simulink model "F16_mod_stock"  (R2024b)
settings: Solver=VariableStepAuto  StartTime=0  StopTime=Tend  RelTol=1e-3
values from neighbouring files (symbols this model uses):
  Param = load_F16_params()    [runF16_mod.m]
libraries: aerolibasang x3, shared6dof x1, aerolibatmos2 x1
settings Model: Creator=sherpa  LastModifiedBy=karth
settings SolverCC: AlgebraicLoopSolver=TrustRegion
settings DataIOCC: SaveFormat=StructureWithTime
settings OptimizationCC: BlockReduction=off  DefaultParameterBehavior=Inlined  OptimizeBlockIOStorage=off  BufferReuse=off
settings DebuggingCC: AlgebraicLoopMsg=none  InitInArrayFormatMsg=none
settings ModelReferenceCC: EnableRefExpFcnMdlSchedulingChecks=on
settings RTWCC: GPUComputeCapability=3.5  DLArmComputeVersion=19.05

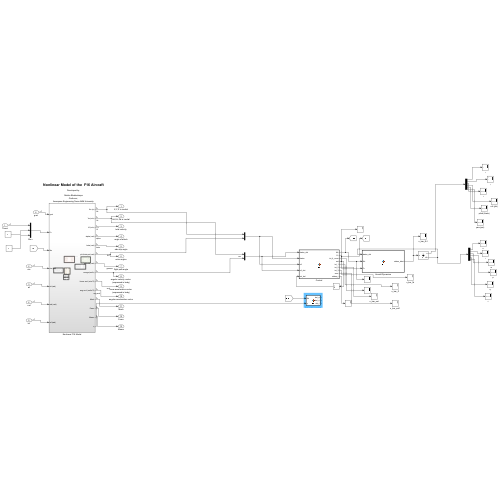
[thumbnail: Simulink's stored preview of the top-level diagram]
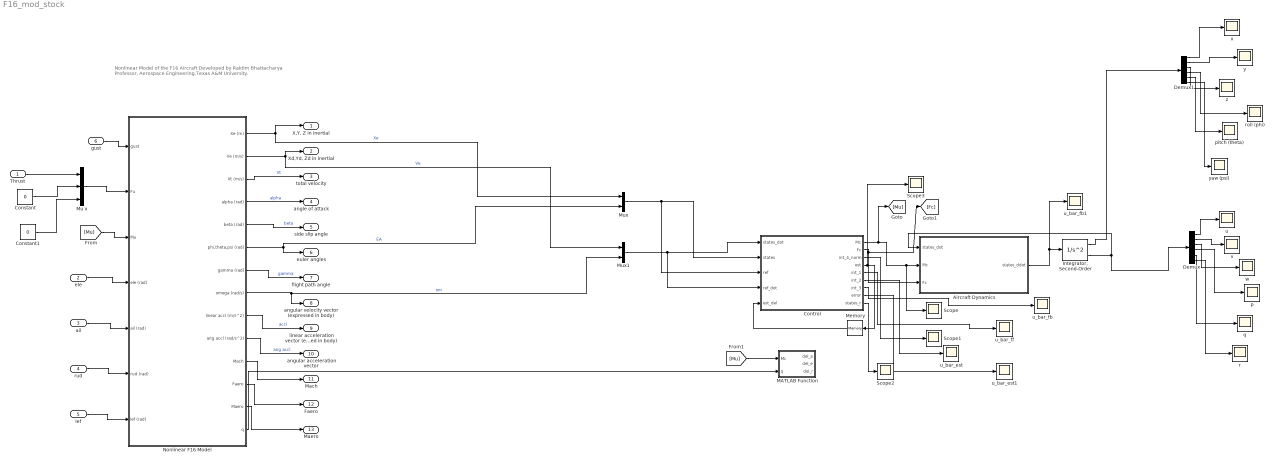
== system F16_mod_stock ==
  note: Nonlinear Model of the F16 Aircraft
      |
      | Developed by
      |
      | Raktim Bhattacharya
      | Professor,
      | Aerospace Engineering,Texas A&M University.
  Thrust : Inport
  ele : Inport  Port=2
  ail : Inport  Port=3
  rud : Inport  Port=4
  lef : Inport  Port=5
  gust : Inport  Port=6
  Aircraft Dynamics : MATLAB Function  TreatAsAtomicUnit=on
  Constant : Constant  Value=0
  Constant1 : Constant  Value=0
  Control : MATLAB Function  TreatAsAtomicUnit=on
  Demux : Demux  Outputs=6
  Demux1 : Demux  Outputs=6
  "Integrator, Second-Order" : SecondOrderIntegrator  ICX=[0;0;0;0;0;0]  ICDXDT=[250;0;0;0;0;0]
  MATLAB Function : MATLAB Function  TreatAsAtomicUnit=on
  Memory : Memory  InitialCondition=[0;0;0]
  Mu x : Mux  Inputs=3
  Mux : Mux  Inputs=2
  Mux1 : Mux  Inputs=2
  Nonlinear F16 Model : Subsystem
  Scope{,1..3} (4 alike) : Scope
  p : Scope
  pitch (theta) : Scope
  q : Scope
  r : Scope
  roll (phi) : Scope
  u : Scope
  u_bar_est : Scope
  u_bar_est1 : Scope
  u_bar_fb : Scope
  u_bar_fb1 : Scope
  u_bar_ff : Scope
  v : Scope
  w : Scope
  x : Scope
  y : Scope
  yaw (psi) : Scope
  z : Scope
  "X,Y, Z in inertial" : Outport
  "Xd,Yd, Zd in inertial" : Outport  Port=2
  total velocity : Outport  Port=3
  angle of attack : Outport  Port=4
  side slip angle : Outport  Port=5
  euler angles : Outport  Port=6
  flight path angle : Outport  Port=7
  angular velocity vector (expressed in body) : Outport  Port=8
  linear acceleration vector (expressed in body) : Outport  Port=9
  angular acceleration vector : Outport  Port=10
  Mach : Outport  Port=11
  Faero : Outport  Port=12
  Maero : Outport  Port=13
  wires:
  Nonlinear F16 Model/1(Xe (m)) -> "X,Y, Z in inertial"/1, Mux/1  "Xe"
  Nonlinear F16 Model/3(Vt (m/s)) -> total velocity/1  "Vt"
  Nonlinear F16 Model/4(alpha (rad)) -> angle of attack/1  "alpha"
  Nonlinear F16 Model/5(beta (rad)) -> side slip angle/1  "beta"
  Nonlinear F16 Model/7(gamma (rad)) -> flight path angle/1  "gamma"
  Nonlinear F16 Model/8(omega (rad/s)) -> angular velocity vector (expressed in body)/1, Mux1/2  "om"
  Nonlinear F16 Model/9(linear accl (m/s^2)) -> linear acceleration vector (expressed in body)/1  "accl"
  Nonlinear F16 Model/6(phi,theta,psi (rad)) -> euler angles/1, Mux/2  "EA"
  Nonlinear F16 Model/2(Ve (m/s)) -> "Xd,Yd, Zd in inertial"/1, Mux1/1  "Ve"
  Nonlinear F16 Model/10(ang accl (rad/s^2)) -> angular acceleration vector/1  "ang accl"
  Nonlinear F16 Model/11(Mach) -> Mach/1
  Thrust/1 -> Mu x/1
  ele/1 -> Nonlinear F16 Model/4(ele (rad))
  rud/1 -> Nonlinear F16 Model/6(rud (rad))
  lef/1 -> Nonlinear F16 Model/7(lef (rad))
  ail/1 -> Nonlinear F16 Model/5(ail (rad))
  gust/1 -> Nonlinear F16 Model/1(gust)
  Nonlinear F16 Model/12(Faero) -> Faero/1
  Nonlinear F16 Model/13(Maero) -> Maero/1
  Demux/3 -> w/1
  Control/7(int_3) -> u_bar_fb/1
  Control/1(Mc) -> [Mu], Scope/1, Aircraft Dynamics/2(Mc)
  Demux1/5 -> pitch (theta)/1
  Control/5(int_1) -> u_bar_ff/1
  Demux/6 -> r/1
  Control/9(states_r) -> Scope2/1
  Control/6(int_2) -> u_bar_est/1
  Aircraft Dynamics/1(states_ddot) -> "Integrator, Second-Order"/1, u_bar_fb1/1
  Demux/1 -> u/1
  Demux1/3 -> z/1
  Demux1/4 -> roll (phi)/1
  Control/3(int_4_norm) -> Scope1/1
  Memory/1 -> Control/5(est_del)
  Demux/2 -> v/1
  Demux/5 -> q/1
  "Integrator, Second-Order"/1 -> Demux1/1
  "Integrator, Second-Order"/2 -> Demux/1, Aircraft Dynamics/1(states_dot)
  Demux1/2 -> y/1
  Control/8(error) -> u_bar_est1/1
  Demux/4 -> p/1
  Demux1/1 -> x/1
  Demux1/6 -> yaw (psi)/1
  Control/4(est) -> Memory/1, Scope3/1
  [Mu] -> Nonlinear F16 Model/3(Mu)
  Control/2(Fc) -> [Fc], Aircraft Dynamics/3(Fc)
  Mux/1 -> Control/3(ref), Control/2(states)
  Mux1/1 -> Control/4(ref_dot), Control/1(states_dot)
  Constant/1 -> Mu x/2
  Mu x/1 -> Nonlinear F16 Model/2(Fu)
  Constant1/1 -> Mu x/3
  Nonlinear F16 Model/14(q) -> MATLAB Function/2(q)
  [Mu] -> MATLAB Function/1(Mc)

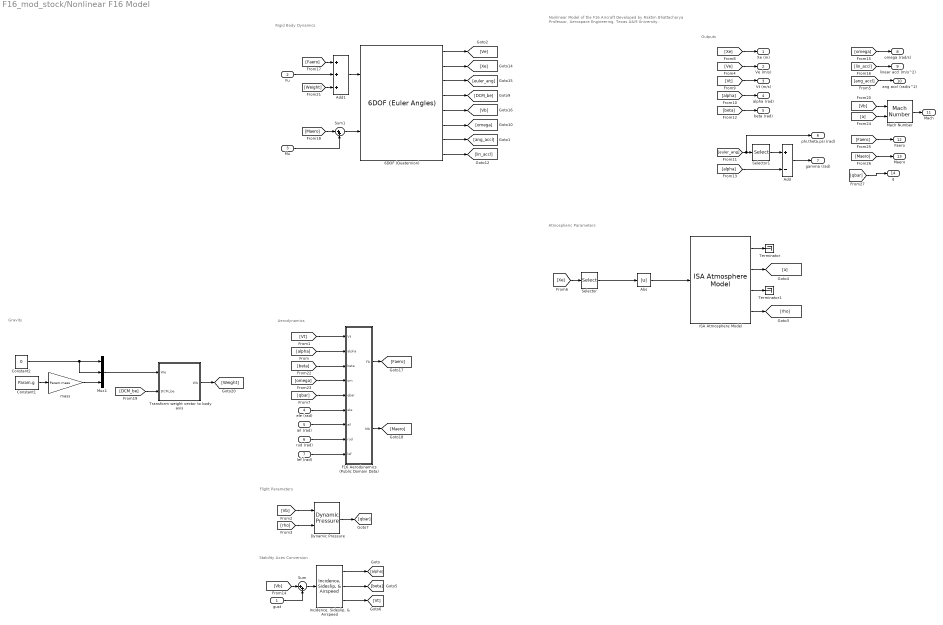
== system F16_mod_stock/Nonlinear F16 Model ==
  note: Gravity
  note: Nonlinear Model of the F16 Aircraft
      |
      | Developed by Raktim Bhattacharya
      | Professor, Aerospace Engineering,
      | Texas A&M University.
  note: Aerodynamics
  note: Outputs
  note: Rigid Body Dynamics
  note: Stability Axes Conversion
  note: Atmospheric Parameters
  note: Flight Parameters
  gust : Inport  PortDimensions=3
  Fu : Inport  Port=2
  Mu : Inport  Port=3  PortDimensions=3
  ele (rad) : Inport  Port=4
  ail (rad) : Inport  Port=5
  rud (rad) : Inport  Port=6
  lef (rad) : Inport  Port=7
  6DOF (Quaternion) : shared6dof/6DOF (Euler Angles)  units=Metric (MKS)  mtype=Fixed  rep=Euler Angles  xme_0=IC.inertial_position  Vm_0=IC.body_velocity  eul_0=IC.euler_angles  pm_0=IC.omega  mass_0=Param.mass  mass_e=0.5  mass_f=2.0  inertia=Param.moi  inertia_e=eye(3)  inertia_f=2*eye(3)  k_quat=1.0  vre_flag=on  abi_flag=off  aMode=0  xme_statename={'Xe', 'Ye', 'Ze'}  Vm_statename={'U', 'v', 'w'}  eul_statename=''  quat_statename={'qr', 'qi', 'qj', 'qk'}  pm_statename={'p', 'q', 'r'}  mass_statename=''
      settings: LibrarySourceBlock=aerolib6dof2/6DOF (Quaternion)
  Abs : Abs  SaturateOnIntegerOverflow=off
  Add : Sum  Inputs=+-
  Add1 : Sum  Inputs=+++
  Constant1 : Constant  Value=Param.g
  Constant2 : Constant  Value=0
  Dynamic Pressure : aerolibasang/Dynamic Pressure
  F16 Aerodynamics (Public Domain Data) : Subsystem
  ISA Atmosphere Model : aerolibatmos2/ISA Atmosphere Model  useExtended=off  action=Warning  custom=off  viscosityOut=off  g=9.80665  gamma=1.4  R=287.0531  L=0.0065  h_trop=11000  h_strat=20000  rho0=1.225  P0=101325  T0=288.15  h0=0  S=110.4  Tref=273.15  muref=1.716e-5
  "Incidence, Sideslip, & Airspeed" : aerolibasang/Incidence, Sideslip, & Airspeed
  Mach Number : aerolibasang/Mach Number
  Mux1 : Mux  Inputs=3
  Selector : Selector  InputPortWidth=3  IndexOptions=Index vector (dialog)  Indices=3  OutputSizes=1
  Selector1 : Selector  InputPortWidth=3  IndexOptions=Index vector (dialog)  Indices=2  OutputSizes=1
  Sum : Sum  Inputs=|++
  Sum1 : Sum  Inputs=|++
  Terminator : Terminator
  Terminator1 : Terminator
  Transform weight vector to body axis : MATLAB Function  TreatAsAtomicUnit=on
  mass : Gain  Gain=Param.mass
  Xe (m) : Outport
  Ve (m/s) : Outport  Port=2
  Vt (m/s) : Outport  Port=3
  alpha (rad) : Outport  Port=4
  beta (rad) : Outport  Port=5
  phi,theta,psi (rad) : Outport  Port=6
  gamma (rad) : Outport  Port=7
  omega (rad/s) : Outport  Port=8
  linear accl (m/s^2) : Outport  Port=9
  ang accl (rad/s^2) : Outport  Port=10
  Mach : Outport  Port=11
  Faero : Outport  Port=12
  Maero : Outport  Port=13
  q : Outport  Port=14
  wires:
  [Xe] -> Selector/1
  [beta] -> beta (rad)/1
  "Incidence, Sideslip, & Airspeed"/3 -> [Vt]
  ISA Atmosphere Model/3 -> Terminator1/1
  ISA Atmosphere Model/1 -> Terminator/1
  ISA Atmosphere Model/4 -> [rho]
  [rho] -> Dynamic Pressure/2
  [lin_accl] -> linear accl (m/s^2)/1
  [alpha] -> alpha (rad)/1
  ISA Atmosphere Model/2 -> [a]
  [Vb] -> Dynamic Pressure/1
  Add/1 -> gamma (rad)/1
  [Vt] -> Vt (m/s)/1
  "Incidence, Sideslip, & Airspeed"/2 -> [beta]
  Selector1/1 -> Add/1
  "Incidence, Sideslip, & Airspeed"/1 -> [alpha]
  Selector/1 -> Abs/1
  [alpha] -> Add/2
  [euler_ang] -> phi,theta,psi (rad)/1, Selector1/1
  [omega] -> omega (rad/s)/1
  Dynamic Pressure/1 -> [qbar]
  [Xe] -> Xe (m)/1
  Constant1/1 -> mass/1
  mass/1 -> Mux1/3
  Mux1/1 -> Transform weight vector to body axis/1(We)
  Transform weight vector to body axis/1(Wb) -> [Weight]
  [DCM_be] -> Transform weight vector to body axis/2(DCM_be)
  Constant2/1 -> Mux1/2, Mux1/1
  [Faero] -> Add1/1
  Fu/1 -> Add1/2
  [Weight] -> Add1/3
  Add1/1 -> 6DOF (Quaternion)/1
  [Vb] -> Sum/1
  Sum/1 -> "Incidence, Sideslip, & Airspeed"/1
  gust/1 -> Sum/2
  [Maero] -> Sum1/1
  Mu/1 -> Sum1/2
  6DOF (Quaternion)/1 -> [Ve]
  6DOF (Quaternion)/2 -> [Xe]
  6DOF (Quaternion)/3 -> [euler_ang]
  6DOF (Quaternion)/4 -> [DCM_be]
  6DOF (Quaternion)/5 -> [Vb]
  6DOF (Quaternion)/6 -> [omega]
  6DOF (Quaternion)/7 -> [ang_accl]
  6DOF (Quaternion)/8 -> [lin_accl]
  [Ve] -> Ve (m/s)/1
  [ang_accl] -> ang accl (rad/s^2)/1
  [Vb] -> Mach Number/1
  [a] -> Mach Number/2
  Mach Number/1 -> Mach/1
  F16 Aerodynamics (Public Domain Data)/1(Fb) -> [Faero]
  Sum1/1 -> 6DOF (Quaternion)/2
  F16 Aerodynamics (Public Domain Data)/2(Mb) -> [Maero]
  [Vt] -> F16 Aerodynamics (Public Domain Data)/1(Vt)
  [alpha] -> F16 Aerodynamics (Public Domain Data)/2(alpha)
  [beta] -> F16 Aerodynamics (Public Domain Data)/3(beta)
  [omega] -> F16 Aerodynamics (Public Domain Data)/4(om)
  [qbar] -> F16 Aerodynamics (Public Domain Data)/5(qbar)
  ele (rad)/1 -> F16 Aerodynamics (Public Domain Data)/6(ele)
  ail (rad)/1 -> F16 Aerodynamics (Public Domain Data)/7(ail)
  rud (rad)/1 -> F16 Aerodynamics (Public Domain Data)/8(rud)
  lef (rad)/1 -> F16 Aerodynamics (Public Domain Data)/9(lef)
  Abs/1 -> ISA Atmosphere Model/1
  [Faero] -> Faero/1
  [Maero] -> Maero/1
  [qbar] -> q/1

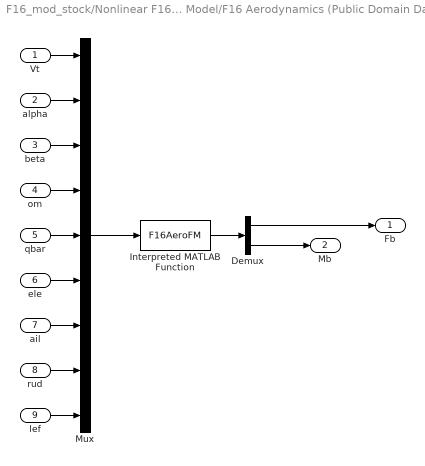
== system F16_mod_stock/Nonlinear F16 Model/F16 Aerodynamics (Public Domain Data) ==
  Vt : Inport
  alpha : Inport  Port=2
  beta : Inport  Port=3
  om : Inport  Port=4
  qbar : Inport  Port=5
  ele : Inport  Port=6
  ail : Inport  Port=7
  rud : Inport  Port=8
  lef : Inport  Port=9
  Demux : Demux  Outputs=2
  Interpreted MATLAB Function : MATLABFcn  MATLABFcn=F16AeroFM  OutputDimensions=6
  Mux : Mux  Inputs=9
  Fb : Outport  PortDimensions=3
  Mb : Outport  Port=2  PortDimensions=3
  wires:
  om/1 -> Mux/4
  beta/1 -> Mux/3
  qbar/1 -> Mux/5
  alpha/1 -> Mux/2
  ele/1 -> Mux/6
  Vt/1 -> Mux/1
  ail/1 -> Mux/7
  rud/1 -> Mux/8
  lef/1 -> Mux/9
  Mux/1 -> Interpreted MATLAB Function/1
  Demux/1 -> Fb/1
  Demux/2 -> Mb/1
  Interpreted MATLAB Function/1 -> Demux/1

== matlab function F16_mod_stock/Nonlinear F16 Model/Transform weight vector to body axis ==
  data: We input; Wb output; DCM_be input
function Wb = fcn(We,DCM_be)
Wb = DCM_be*We; % Weight in body coordinate system. DCM_be is correct, no need for transpose. They must have fixed it in this version.

== matlab function F16_mod_stock/Aircraft Dynamics ==
  data: states_dot input; states_ddot output; Mc input; Fc input
function states_ddot  = fcn(states_dot,Mc,Fc)

% phi, theta , psi == roll_rate, pitch_rate, yaw_rate
theta = 0; % Placeholder angle (pitch) in radians
phi = 0; 

m_aircraft = 24000;
l_aircraft = 17.2;
wingspan = 11.8;
wing_area = 39.9;
wing_width = 4.4;
m_load = 1000;
r_load = 0.3;
n = 4;
wing_mass = 0.12 * m_aircraft;  % this is the combined mass of both wings
r_fuselage = 1.5;
wingspan_new = wingspan - r_fuselage *  2;
m_sym = m_aircraft + n * m_load;
m_asym = m_aircraft + (n-1) * m_load;
%m_aircraft_prime = m_aircraft - m_load; % KR

I_fuselage_origin = 0.5 * (m_aircraft - wing_mass) * r_fuselage.^2;
I_wings = 2 * (1/12) * (wing_mass) * (2 * wing_width.^2);
I_load = n * ((0.5 * m_load * r_load.^2) + (m_load * wing_width.^2));
I_sym = I_fuselage_origin + I_wings + I_load;
cg_x_sym = 0;
cg_y_sym = 0;
cg_z_sym = 0;
cg_shift = (m_aircraft * 0 + (n/2)*m_load - (n/2-1)*m_load)/m_asym;
g = 9.81000;

I_xx_asym = 1.5e4; 
I_yy_asym = 2.0e4;
I_zz_asym = 2.5e4;
I_asym = diag([I_xx_asym, I_yy_asym, I_zz_asym]); % Diagonal terms (kg·m²)

I_xz_asym = 0.02 * I_xx_asym; % Small cross-term (2% of I_xx)
I_yz_asym = 0.02 * I_yy_asym; 
I_xy_asym = 0.02 * I_zz_asym; 

%I_prime = 0; % KR

Zcm = 0.1; 
Ycm = 0.2;
Xcm = 0.15;

% theta = [p q r]^T
% omega = [u v w]^T

p = states_dot(1);
q = states_dot(2);
r = states_dot(3);
u = states_dot(4);
v = states_dot(5);
w = states_dot(6);

Ms = [0;0;0];
Fx = 0;
Fy = 0;
Fz = 0;
Fs = [Fx;Fy;Fz];

A = [0 -m_asym*Zcm m_asym*Ycm; m_asym*Zcm 0 -m_asym*Xcm; -m_asym*Ycm m_asym*Xcm 0];

F1_t = -(q*w) + r*v + (q.^2 + r.^2)*Xcm - (p*q*Ycm) - (r*p*Zcm) + (1/m_asym)*Fx;
F2_t = -(r*u) + p*w + (r.^2 + p.^2)*Ycm - (p*q*Xcm) - (q*r*Zcm) + (1/m_asym)*Fy;
F3_t = -(p*v) + q*u + (p.^2 + q.^2)*Zcm - (r*p*Xcm) - q*r*Ycm + (1/m_asym)*Fz;
F=[F1_t;F2_t;F3_t];

M1_t = I_xz_asym*p*q + (I_yy_asym-I_zz_asym)*q*r - I_xy_asym*r*p + I_yz_asym*(q.^2-r.^2) + m_asym*(q*u - p*v)*Ycm + m_asym*(r*u-p*w)*Zcm + (-Zcm)*m_asym*g*cos(theta)*sin(phi) + Ycm*m_asym*g*cos(theta)*cos(phi);
M2_t = (-I_yz_asym)*p*q + I_xy_asym*q*r + (I_zz_asym-I_xx_asym)*r*p + I_xz_asym*(r.^2-p.^2) + m_asym*(p*v - q*u)*Xcm + m_asym*(r*v-q*w)*Zcm + (-Zcm)*m_asym*g*sin(theta) - Xcm*m_asym*g*cos(theta)*cos(phi);
M3_t = (I_xx_asym-I_yy_asym)*p*q - I_xz_asym*q*r - I_yz_asym*r*p + I_xy_asym*(p.^2-q.^2) + m_asym*(p*w - r*u)*Xcm + m_asym*(q*w-r*v)*Ycm + Ycm*m_asym*g*sin(theta) + Xcm*m_asym*g*cos(theta)*sin(phi);

Mi = [M1_t;M2_t;M3_t];

Fx = Fc(1);
Fy = Fc(2);
Fz = Fc(3);

u_dot = -q*w + r*v - g*sin(theta) + (1/m_sym)*Fx;
v_dot = -r*u + p*w + g*cos(theta)*sin(phi) + (1/m_sym)*Fy;
w_dot = -p*v + q*u + g*cos(theta)*cos(phi) + (1/m_sym)*Fz;

theta_dot = inv((1/m_asym)* (A^2) + I_asym) * (-A*F - (1/m_asym)*A*Fs +  Mi + Ms + Mc);
omega_dot = [u_dot;v_dot;w_dot];
states_ddot  = [omega_dot;theta_dot];

== matlab function F16_mod_stock/Control ==
  data: states_dot input; states input; Mc output; ref input; Fc output; int_4_norm output; ref_dot input; est output; est_del input; int_1 output; int_2 output; int_3 output; error output; states_r output
function [Mc,Fc,int_4_norm,est, int_1, int_2, int_3,error, states_r] = fcn(states_dot,states,ref,ref_dot,est_del)

states_r = states(4:6);
states_r_dot = states_dot(4:6);
ref_r = ref(4:6);
ref_r_dot = ref_dot(4:6);

error = states_r - ref_r;
error_dot = states_r_dot - ref_r_dot;

theta = 0; % Placeholder angle (pitch) in radians
phi = 0; 

m_aircraft = 24000;
l_aircraft = 17.2;
wingspan = 9.144;
wing_area = 39.9;
wing_width = 4.4;
m_load = 1000;
r_load = 0.3;
n = 4;
wing_mass = 0.12 * m_aircraft;  % this is the combined mass of both wings
r_fuselage = 1.5;
wingspan_new = wingspan - r_fuselage *  2;
m_sym = m_aircraft + n * m_load;
m_asym = m_aircraft + (n-1) * m_load;
m_aircraft_prime = m_aircraft - m_load; % KR

I_fuselage_origin = 0.5 * (m_aircraft - wing_mass) * r_fuselage.^2;
I_wings = 2 * (1/12) * (wing_mass) * (2 * wing_width.^2);
I_load = n * ((0.5 * m_load * r_load.^2) + (m_load * wing_width.^2));
I_sym = I_fuselage_origin + I_wings + I_load;
cg_x_sym = 0;
cg_y_sym = 0;
cg_z_sym = 0;
cg_shift = (m_aircraft * 0 + (n/2)*m_load - (n/2-1)*m_load)/m_asym;
g = 9.81000;

I_asym = diag([1.5e4, 2.0e4, 2.5e4]); % Diagonal terms (kg·m²)
I_xx_asym = 1.5e4; 
I_yy_asym = 2.0e4;
I_zz_asym = 2.5e4;

I_xz_asym = 0.02 * I_xx_asym; % Small cross-term (2% of I_xx)
I_yz_asym = 0.02 * I_yy_asym; 
I_xy_asym = 0.02 * I_zz_asym; 

I_prime = 0; %KR

Zcm = 0.1; 
Ycm = 0.2;
Xcm = 0.15;

Fx = 0;
Fy = 0;
Fz = 0;
Fs = [Fx;
     Fy;
     Fz];

Ms = [0;0;0];
Mxs = Ms(1);
Mys = Ms(2);
Mzs = Ms(3);

p = states_dot(1);
q = states_dot(2);
r = states_dot(3);
u = states_dot(4);
v = states_dot(5);
w = states_dot(6);

M = [
    1 0 0 0 Zcm -Ycm; 
    0 1 0 -Zcm 0 Xcm; 
    0 0 1 Ycm -Xcm 0; 
    0 -m_asym*Zcm m_asym*Ycm I_xx_asym -I_xy_asym -I_xz_asym; 
    m_asym*Zcm 0 -m_asym*Xcm -I_xy_asym I_yy_asym -I_yz_asym; 
    -m_asym*Ycm m_asym*Xcm 0 -I_xz_asym -I_yz_asym I_zz_asym
    ];

% S_dot = [
%     u_dot; 
%     v_dot; 
%     w_dot; 
%     p_dot; 
%     q_dot; 
%     r_dot
%     ];

C = [
    -q*w + r*v + (q.^2 + r.^2)*Xcm - p*q*Ycm - r*p*Zcm;
    -r*u + p*w + (r.^2 + p.^2)*Ycm - p*q*Xcm - q*r*Zcm;
    -p*v + q*u + (p.^2 + q.^2)*Zcm - r*p*Xcm - q*r*Ycm;
    I_xz_asym*p*q + (I_yy_asym-I_zz_asym)*q*r - I_xy_asym*r*p + I_yz_asym*(q.^2-r.^2) + m_sym*(q*u - p*v)*Ycm + m_sym*(r*u-p*w)*Zcm;
    (-I_yz_asym)*p*q + I_xy_asym*q*r - (I_zz_asym-I_xx_asym)*r*p + I_xz_asym*(r.^2-p.^2) + m_sym*(p*v - q*u)*Xcm + m_sym*(r*v-q*w)*Zcm;
    (I_xx_asym-I_yy_asym)*p*q - I_xz_asym*q*r - I_yz_asym*r*p + I_xy_asym*(p.^2-q.^2) + m_sym*(p*w - r*u)*Xcm + m_sym*(q*w-r*v)*Ycm
    ];

% A = [
%     -g*sin(theta);
%     g*cos(theta)*sin(phi);
%     g*cos(theta)*cos(phi);
%     (-Zcm)*m_sym*g*cos(theta)*sin(phi) + Ycm*m_sym*g*cos(theta)*cos(phi);
%     (-Zcm)*m_sym*g*sin(theta) - Xcm*m_sym*g*cos(theta)*cos(phi);
%     Ycm*m_sym*g*sin(theta) + Xcm*m_sym*g*cos(theta)*sin(phi)
%     ];

A = [0 -m_asym*Zcm m_asym*Ycm; m_asym*Zcm 0 -m_asym*Xcm; -m_asym*Ycm m_asym*Xcm 0];

D = [
    (1/m_sym) 0 0 0 0 0;
    0 (1/m_sym) 0 0 0 0;
    0 0 (1/m_sym) 0 0 0;
    0 0 0 1 0 0;
    0 0 0 0 1 0;
    0 0 0 0 0 1
    ];

% U = [
%     Fx;
%     Fy;
%     Fz;
%     Mx;
%     My;
%     Mz
%     ];

% S_dot = inv(M) * (C + A) + inv(M) * D * U;

%F1_t = -q*w + r*v + (q.^2 + r.^2)*Xcm - p*q*Ycm - r*p*Zcm + (1/m_asym)*Fx;
%F2_t = -r*u + p*w + (r.^2 + p.^2)*Ycm - p*q*Xcm - q*r*Zcm + (1/m_asym)*Fy;
%F3_t = -p*v + q*u + (p.^2 + q.^2)*Zcm - r*p*Xcm - q*r*Ycm + (1/m_asym)*Fz;
%F = [F1_t;F2_t;F3_t];


F1_t = -q*w + r*v + (q.^2 + r.^2)*Xcm - p*q*Ycm - r*p*Zcm + (1/m_asym)*Fx;
F2_t = -r*u + p*w + (r.^2 + p.^2)*Ycm - p*q*Xcm - q*r*Zcm + (1/m_asym)*Fy;
F3_t = -p*v + q*u + (p.^2 + q.^2)*Zcm - r*p*Xcm - q*r*Ycm + (1/m_asym)*Fz;
F=[F1_t;F2_t;F3_t];

%M1_t = I_xz_asym*p*q + (I_yy_asym-I_zz_asym)*q*r - I_xy_asym*r*p + I_yz_asym*(q.^2-r.^2) + m_asym*(q*u - p*v)*Ycm + m_asym*(r*u-p*w)*Zcm + (-Zcm)*m_asym*g*cos(theta)*sin(phi) + Ycm*m_asym*g*cos(theta)*cos(phi);
%M2_t = (-I_yz_asym)*p*q + I_xy_asym*q*r - (I_zz_asym-I_xx_asym)*r*p + I_xz_asym*(r.^2-p.^2) + m_asym*(p*v - q*u)*Xcm + m_asym*(r*v-q*w)*Zcm + (-Zcm)*m_asym*g*sin(theta) - Xcm*m_asym*g*cos(theta)*cos(phi);
%M3_t = (I_xx_asym-I_yy_asym)*p*q - I_xz_asym*q*r - I_yz_asym*r*p + I_xy_asym*(p.^2-q.^2) + m_asym*(p*w - r*u)*Xcm + m_asym*(q*w-r*v)*Ycm + Ycm*m_asym*g*sin(theta) + Xcm*m_asym*g*cos(theta)*sin(phi);
%Mi = [M1_t; M2_t; M3_t];

M1_t = I_xz_asym*p*q + (I_yy_asym-I_zz_asym)*q*r - I_xy_asym*r*p + I_yz_asym*(q.^2-r.^2) + m_asym*(q*u - p*v)*Ycm + m_asym*(r*u-p*w)*Zcm + (-Zcm)*m_asym*g*cos(theta)*sin(phi) + Ycm*m_asym*g*cos(theta)*cos(phi);
M2_t = (-I_yz_asym)*p*q + I_xy_asym*q*r + (I_zz_asym-I_xx_asym)*r*p + I_xz_asym*(r.^2-p.^2) + m_asym*(p*v - q*u)*Xcm + m_asym*(r*v-q*w)*Zcm + (-Zcm)*m_asym*g*sin(theta) - Xcm*m_asym*g*cos(theta)*cos(phi);
M3_t = (I_xx_asym-I_yy_asym)*p*q - I_xz_asym*q*r - I_yz_asym*r*p + I_xy_asym*(p.^2-q.^2) + m_asym*(p*w - r*u)*Xcm + m_asym*(q*w-r*v)*Ycm + Ycm*m_asym*g*sin(theta) + Xcm*m_asym*g*cos(theta)*sin(phi);
Mi = [M1_t; M2_t; M3_t];



int_1 = -A*(F);          % KR
int_2 = -A*(Fs)/m_asym; % KR
int_3 = Mi + Ms; % KR
int_4 = ((1/m_asym)*(A^2)) + I_asym; % KR

fs = inv(int_4) * (int_1 + int_2 + int_3); %KR

gs = (((A^2/m_asym) + I_asym)); %KR Does Myc and Mzc also have to be included in the function definition above?

int_4_norm = norm(int_4,2);
gs_norm = norm(gs,2);

K = diag([10;10;10]);

u_bar_ff = -inv(gs)*(fs);

u_bar_est = inv(gs)*(est_del);

u_bar_fb = -inv(gs)*(K*error);

u_bar = inv(gs)*(-fs - est_del - (K*error));  %ffffffhgb

Fc = [0;0;0];
Mc = u_bar;

est = states_r_dot - fs - ((gs)*u_bar);

== matlab function F16_mod_stock/MATLAB Function ==
  data: del_a output; del_e output; del_r output; Mc input; q input
function [del_a, del_e, del_r] = fcn (Mc, q)

allocation_matrix = [q*S*b*C_l_del_a  q*S*b*C_l_del_e  q*S*b*C_l_del_a  ;
                        0             q*S*c*C_m_del_e        0          ;
                     q*S*b*C_n_del_a  q*S*b*C_n_del_e  q*S*b*C_n_del_a  ;
    ];


inter = allocation_matrix / Mc;
del_a = inter(0);
del_e = inter(1);
del_r = inter(2);
